simulink model "IMFaults"  (R2025b)
settings: Solver=ode23t  StartTime=0.0  StopTime=20  MaxStep=1e-4  RelTol=1e-3  EnableMultiTasking=on
undefined symbols (not defined in the file or in its folder): DELTA_A, DELTA_B, DELTA_C, V_phase
libraries: ee_lib x13, nesl_utility x10, fl_lib x9
CloseFcn:
  | clear simlog_IMStarting
  | clear logsout_IMStarting
Description:
  | Three-Phase Asynchronous Machine Starting
settings Model: Creator=The MathWorks, Inc.  LastModifiedBy=Hp Probook
settings SolverCC: AlgebraicLoopSolver=TrustRegion  MaxZcPerStep=1.0
settings DataIOCC: LimitDataPoints=on  MaxDataPoints=90000  SaveFormat=Array  ReturnWorkspaceOutputs=off
settings OptimizationCC: ReuseModelBlockBuffer=off  LifeSpan=inf
settings DebuggingCC: UnconnectedInputMsg=warning  UnconnectedOutputMsg=warning  UnconnectedLineMsg=warning  SFUnexpectedBacktrackingDiag=warning  SFNoUnconditionalDefaultTransitionDiag=warning  SFExecutionAtInitializationDiag=none  ArithmeticOperatorsInVariantConditions=warning
settings HardwareCC: ProdBitPerPointer=32.0  ProdBitPerSizeT=32.0  ProdBitPerPtrDiffT=32.0  ProdLargestAtomicFloat=None  ProdIntDivRoundTo=Undefined  ProdEndianess=Unspecified  ProdWordSize=32.0  ProdHWDeviceType=32-bit Generic
settings ModelReferenceCC: EnableRefExpFcnMdlSchedulingChecks=on  PropagateSignalLabelsOutOfModel=off
settings SFSimCC: SimUseLocalCustomCode=off  CustomCodeUndefinedFunction=UseInterfaceOnly
settings RTWCC: RTWUseLocalCustomCode=off  GPUComputeCapability=3.5  DLArmComputeVersion=19.05
settings CodeAppCC: StateflowObjectComments=on
settings GRTTargetCC: TargetLangStandard=C89/C90 (ANSI)
settings ConfigComp: CovMetricSettings=dw  CovSaveCumulativeToWorkspaceVar=on  CovSaveSingleToWorkspaceVar=on  CovExternalEMLEnable=off  CovSFcnEnable=off
settings SimscapeCC: SimscapeLogType=all  SimscapeLogSimulationStatistics=on  SimscapeLogName=simlog_IMStarting  SimscapeLogDataHistory=90000.0

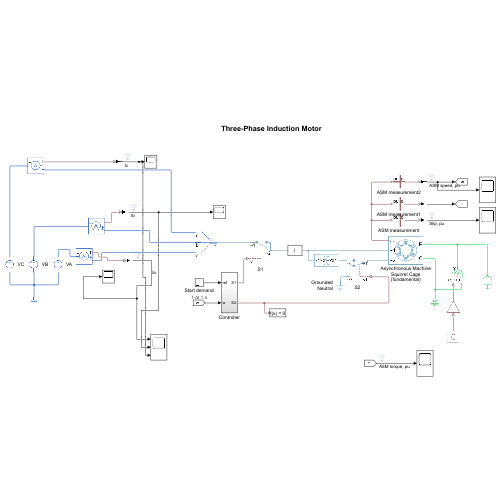
[thumbnail: Simulink's stored preview of the top-level diagram]
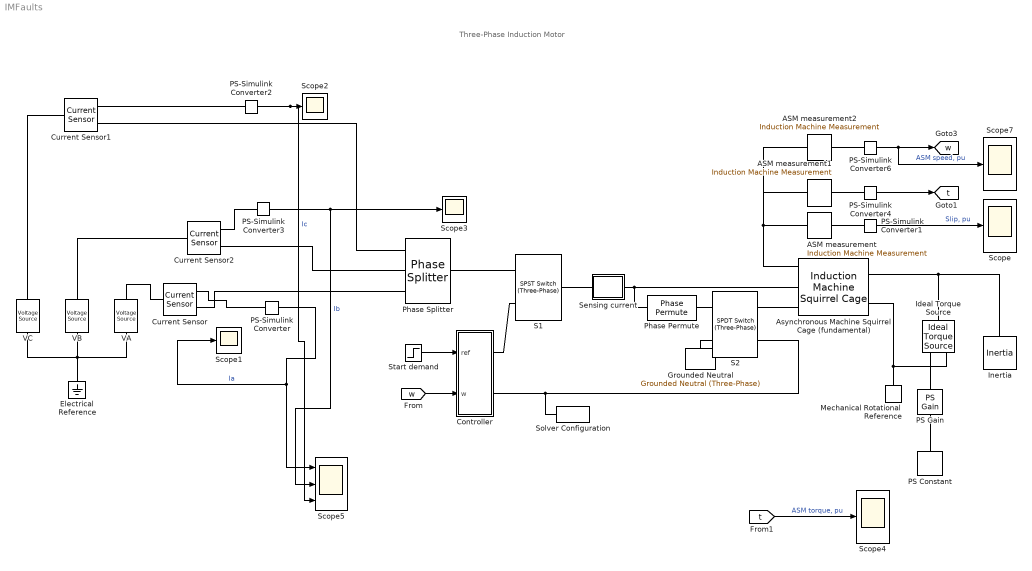
== system IMFaults ==
  note: Three-Phase Induction Motor
  ASM measurement : ee_lib/Electromechanical/Asynchronous/Induction Machine Measurement  output_idx=9
      settings: InternalSimscapePortConfiguration="{\"Bottom\":[],\"Left\":[{\"id\":\"pu_input\",\"label\":\"pu\",\"type\":\"input\"}],\"Right\":[{\"id\":\"pu_output\",\"label\":\"o\",\"type\":\"output\"}],\"Top\":[]}"
  ASM measurement1 : ee_lib/Electromechanical/Asynchronous/Induction Machine Measurement  output_idx=1
      settings: InternalSimscapePortConfiguration="{\"Bottom\":[],\"Left\":[{\"id\":\"pu_input\",\"label\":\"pu\",\"type\":\"input\"}],\"Right\":[{\"id\":\"pu_output\",\"label\":\"o\",\"type\":\"output\"}],\"Top\":[]}"
  ASM measurement2 : ee_lib/Electromechanical/Asynchronous/Induction Machine Measurement  output_idx=2
      settings: InternalSimscapePortConfiguration="{\"Bottom\":[],\"Left\":[{\"id\":\"pu_input\",\"label\":\"pu\",\"type\":\"input\"}],\"Right\":[{\"id\":\"pu_output\",\"label\":\"o\",\"type\":\"output\"}],\"Top\":[]}"
  Asynchronous Machine Squirrel Cage (fundamental) : ee_lib/Electromechanical/Asynchronous/Induction Machine Squirrel Cage  port_option=ee.enum.threePhasePort.composite  SRated=15e3 V*A  VRated=220 V  FRated=60 Hz  nPolePairs=1  param_unit=ee.enum.unit.pu  squirrel_cage=ee.enum.squirrelcage.Single  zero_sequence=ee.enum.park.zerosequence.include  initialization_option=ee.enum.asm.initialization.fluxvariables  Rs=0.25 Ohm  Xls=0.4 Ohm  pu_Rs=0.0258  pu_Lls=0.0413  Rrd=0.14 Ohm  Xlrd=0.41 Ohm  pu_Rrd=0.0145  pu_Llrd=0.0424  Rrd1=0.28 Ohm  Xlrd1=0.82 Ohm  Rrd2=0.28 Ohm  Xlrd2=0.82 Ohm  pu_Rrd1=0.0290  pu_Llrd1=0.0848  pu_Rrd2=0.0290  pu_Llrd2=0.0848  Xm=17 Ohm  pu_Lm=1.7562  X0=0.4 Ohm  pu_L0=0.0413  saturation_option=ee.enum.saturation.include  saturation_i=[0, 4, 9, 18, 25, 34, 50, 68, 95, 120] A  saturation_v=[0, 88, 154, 198, 220, 242, 264, 286, 308, 327] V  pu_saturation_i=[0, .176, .396, .792, 1.1, 1.496, 2.2, 2.992, 4.18, 5.28]  pu_saturation_v=[0, .4, .7, .9, 1, 1.1, 1.2, 1.3, 1.4, 1.4864]  connection_option=ee.enum.Connection.delta1  angular_position_specify=off  angular_position_priority=None  angular_position=0 deg  angular_position_nominal_specify=off  angular_position_nominal_value=1  angular_position_nominal_unit=deg  pu_psids_specify=off  pu_psids_priority=None  pu_psids=0  pu_psids_nominal_specify=off  pu_psids_nominal_value=1  pu_psids_nominal_unit=1  pu_psiqs_specify=off  pu_psiqs_priority=None  pu_psiqs=0  pu_psiqs_nominal_specify=off  pu_psiqs_nominal_value=1  pu_psiqs_nominal_unit=1  pu_psi0s_specify=off  pu_psi0s_priority=None  pu_psi0s=0  pu_psi0s_nominal_specify=off  pu_psi0s_nominal_value=1  pu_psi0s_nominal_unit=1  pu_psidr_specify=off  pu_psidr_priority=None  pu_psidr=0  pu_psidr_nominal_specify=off  pu_psidr_nominal_value=1  pu_psidr_nominal_unit=1  pu_psiqr_specify=off  pu_psiqr_priority=None  pu_psiqr=0  pu_psiqr_nominal_specify=off  pu_psiqr_nominal_value=1  pu_psiqr_nominal_unit=1  pu_psidr1_specify=off  pu_psidr1_priority=None  pu_psidr1=0  pu_psidr1_nominal_specify=off  pu_psidr1_nominal_value=1  pu_psidr1_nominal_unit=1  pu_psiqr1_specify=off  pu_psiqr1_priority=None  pu_psiqr1=0  pu_psiqr1_nominal_specify=off  pu_psiqr1_nominal_value=1  pu_psiqr1_nominal_unit=1  pu_psidr2_specify=off  pu_psidr2_priority=None  pu_psidr2=0  pu_psidr2_nominal_specify=off  pu_psidr2_nominal_value=1  pu_psidr2_nominal_unit=1  pu_psiqr2_specify=off  pu_psiqr2_priority=None  pu_psiqr2=0  pu_psiqr2_nominal_specify=off  pu_psiqr2_nominal_value=1  pu_psiqr2_nominal_unit=1  psids_specify=off  psids_priority=None  psids=0 Wb  psids_nominal_specify=off  psids_nominal_value=1  psids_nominal_unit=Wb  psiqs_specify=off  psiqs_priority=None  psiqs=0 Wb  psiqs_nominal_specify=off  psiqs_nominal_value=1  psiqs_nominal_unit=Wb  psi0s_specify=off  psi0s_priority=None  psi0s=0 Wb  psi0s_nominal_specify=off  psi0s_nominal_value=1  psi0s_nominal_unit=Wb  psidr_specify=off  psidr_priority=None  psidr=0 Wb  psidr_nominal_specify=off  psidr_nominal_value=1  psidr_nominal_unit=Wb  psiqr_specify=off  psiqr_priority=None  psiqr=0 Wb  psiqr_nominal_specify=off  psiqr_nominal_value=1  psiqr_nominal_unit=Wb  psidr1_specify=off  psidr1_priority=None  psidr1=0 Wb  psidr1_nominal_specify=off  psidr1_nominal_value=1  psidr1_nominal_unit=Wb  psiqr1_specify=off  psiqr1_priority=None  psiqr1=0 Wb  psiqr1_nominal_specify=off  psiqr1_nominal_value=1  psiqr1_nominal_unit=Wb  psidr2_specify=off  psidr2_priority=None  psidr2=0 Wb  psidr2_nominal_specify=off  psidr2_nominal_value=1  psidr2_nominal_unit=Wb  psiqr2_specify=off  psiqr2_priority=None  psiqr2=0 Wb  psiqr2_nominal_specify=off  psiqr2_nominal_value=1  psiqr2_nominal_unit=Wb  slip_specify=off  slip_priority=None  slip=0  slip_nominal_specify=off  slip_nominal_value=1  slip_nominal_unit=1  real_power_generated_specify=off  real_power_generated_priority=None  real_power_generated=0 W  real_power_generated_nominal_specify=off  real_power_generated_nominal_value=1  real_power_generated_nominal_unit=W  mechanical_power_consumed_specify=off  mechanical_power_consumed_priority=None  mechanical_power_consumed=0 W  mechanical_power_consumed_nominal_specify=off  mechanical_power_consumed_nominal_value=1  mechanical_power_consumed_nominal_unit=W  Tmeas=298.15 K  alpha=3.93e-3 1/K  alpha_cage=4.4e-3 1/K  stator_thermal_mass=100 J/K  rotor_thermal_mass=200 J/K  temperatureA_specify=off  temperatureA_priority=High  temperatureA=25 degC  temperatureA_nominal_specify=off  temperatureA_nominal_value=1  temperatureA_nominal_unit=degC  temperatureB_specify=off  temperatureB_priority=High  temperatureB=25 degC  temperatureB_nominal_specify=off  temperatureB_nominal_value=1  temperatureB_nominal_unit=degC  temperatureC_specify=off  temperatureC_priority=High  temperatureC=25 degC  temperatureC_nominal_specify=off  temperatureC_nominal_value=1  temperatureC_nominal_unit=degC  temperatureR_specify=off  temperatureR_priority=High  temperatureR=25 degC  temperatureR_nominal_specify=off  temperatureR_nominal_value=1  temperatureR_nominal_unit=degC
      settings: InternalSimscapePortConfiguration="{\"Bottom\":[],\"Left\":[{\"id\":\"R\",\"label\":\"R\",\"type\":\"foundation.mechanical.rotational.rotational\"},{\"id\":\"C\",\"label\":\"C\",\"type\":\"foundation.mechanical.rotational.rotational\"}],\"Right\":[{\"id\":\"pu_output\",\"label\":\"pu\",\"type\":\"output\"},{\"id\":\"N1\",\"label\":\"~1\",\"type\":\"foundation.electrical.three_phase\"},{\"id\":\"N2\",\"label\":\"~2\",\"type\":\"foundation.electrical.three_phase\"}],\"Top\":[]}"
  Controller : Subsystem
  Current Sensor : fl_lib/Electrical/Electrical Sensors/Current Sensor
  Current Sensor1 : fl_lib/Electrical/Electrical Sensors/Current Sensor
  Current Sensor2 : fl_lib/Electrical/Electrical Sensors/Current Sensor
  Electrical Reference : fl_lib/Electrical/Electrical Elements/Electrical Reference
  Grounded Neutral : ee_lib/Connectors & References/Grounded Neutral (Three-Phase)
  Ideal Torque Source : fl_lib/Mechanical/Mechanical Sources/Ideal Torque Source
  Inertia : fl_lib/Mechanical/Rotational Elements/Inertia  inertia=0.001 kg*m^2  num_ports=foundation.enum.numPorts2.one  w_specify=off  w_priority=High  w=0 rad/s  w_nominal_specify=off  w_nominal_value=1  w_nominal_unit=rad/s  t_specify=off  t_priority=None  t=0 N*m  t_nominal_specify=off  t_nominal_value=1  t_nominal_unit=N*m
  Mechanical Rotational Reference : fl_lib/Mechanical/Rotational Elements/Mechanical Rotational Reference
  PS Constant : fl_lib/Physical Signals/Sources/PS Constant  constant=10 N*m
  PS Gain : fl_lib/Physical Signals/Functions/PS Gain  gain=-2
  PS-Simulink Converter : nesl_utility/PS-Simulink Converter  PhysicalDomain=network_engine_domain  SubClassName=ps_output  LeftPortType=input  RightPortType=output  PseudoPeriodic=off  Frequencies=[]  VectorFormat=inherit  Unit=inherit  AffineConversion=off
  PS-Simulink Converter1 : nesl_utility/PS-Simulink Converter  PhysicalDomain=network_engine_domain  SubClassName=ps_output  LeftPortType=input  RightPortType=output  PseudoPeriodic=off  Frequencies=[]  VectorFormat=1-D array  Unit=1  AffineConversion=off
  PS-Simulink Converter2 : nesl_utility/PS-Simulink Converter  PhysicalDomain=network_engine_domain  SubClassName=ps_output  LeftPortType=input  RightPortType=output  PseudoPeriodic=off  Frequencies=[]  VectorFormat=inherit  Unit=inherit  AffineConversion=off
  PS-Simulink Converter3 : nesl_utility/PS-Simulink Converter  PhysicalDomain=network_engine_domain  SubClassName=ps_output  LeftPortType=input  RightPortType=output  PseudoPeriodic=off  Frequencies=[]  VectorFormat=inherit  Unit=inherit  AffineConversion=off
  PS-Simulink Converter4 : nesl_utility/PS-Simulink Converter  PhysicalDomain=network_engine_domain  SubClassName=ps_output  LeftPortType=input  RightPortType=output  PseudoPeriodic=off  Frequencies=[]  VectorFormat=1-D array  Unit=1  AffineConversion=off
  PS-Simulink Converter6 : nesl_utility/PS-Simulink Converter  PhysicalDomain=network_engine_domain  SubClassName=ps_output  LeftPortType=input  RightPortType=output  PseudoPeriodic=off  Frequencies=[]  VectorFormat=1-D array  Unit=1  AffineConversion=off
  Phase Permute : ee_lib/Connectors & References/Phase Permute
      settings: InternalSimscapePortConfiguration="{\"Bottom\":[],\"Left\":[{\"id\":\"N123\",\"label\":\"~123\",\"type\":\"foundation.electrical.three_phase\"}],\"Right\":[{\"id\":\"N231\",\"label\":\"~231\",\"type\":\"foundation.electrical.three_phase\"}],\"Top\":[]}"
  Phase Splitter : ee_lib/Connectors & References/Phase Splitter
  S1 : ee_lib/Switches & Breakers/SPST Switch (Three-Phase)  R_closed=0.001 Ohm  G_open=1e-6 1/Ohm  threshold=0.5 V  i_vT_specify=off  i_vT_priority=None  i_vT=0 A  i_vT_nominal_specify=off  i_vT_nominal_value=1  i_vT_nominal_unit=A  I_specify=off  I_priority=None  I=[ 0 0 0 ] A  I_nominal_specify=off  I_nominal_value=1  I_nominal_unit=A  V_specify=off  V_priority=None  V=[ 0 0 0 ] V  V_nominal_specify=off  V_nominal_value=1  V_nominal_unit=V  i_a_specify=off  i_a_priority=None  i_a=0 A  i_a_nominal_specify=off  i_a_nominal_value=1  i_a_nominal_unit=A  v_a_specify=off  v_a_priority=None  v_a=0 V  v_a_nominal_specify=off  v_a_nominal_value=1  v_a_nominal_unit=V  i_b_specify=off  i_b_priority=None  i_b=0 A  i_b_nominal_specify=off  i_b_nominal_value=1  i_b_nominal_unit=A  v_b_specify=off  v_b_priority=None  v_b=0 V  v_b_nominal_specify=off  v_b_nominal_value=1  v_b_nominal_unit=V  i_c_specify=off  i_c_priority=None  i_c=0 A  i_c_nominal_specify=off  i_c_nominal_value=1  i_c_nominal_unit=A  v_c_specify=off  v_c_priority=None  v_c=0 V  v_c_nominal_specify=off  v_c_nominal_value=1  v_c_nominal_unit=V
      settings: InternalSimscapePortConfiguration="{\"Bottom\":[],\"Left\":[{\"id\":\"vT\",\"label\":\"vT\",\"type\":\"input\"},{\"id\":\"N1\",\"label\":\"~1\",\"type\":\"foundation.electrical.three_phase\"}],\"Right\":[{\"id\":\"N2\",\"label\":\"~2\",\"type\":\"foundation.electrical.three_phase\"}],\"Top\":[]}"
  S2 : ee_lib/Switches & Breakers/SPDT Switch (Three-Phase)  R_closed=0.001 Ohm  G_open=1e-6 1/Ohm  threshold=0.5 V  i_vT_specify=off  i_vT_priority=None  i_vT=0 A  i_vT_nominal_specify=off  i_vT_nominal_value=1  i_vT_nominal_unit=A  I12_specify=off  I12_priority=None  I12=[ 0 0 0 ] A  I12_nominal_specify=off  I12_nominal_value=1  I12_nominal_unit=A  V12_specify=off  V12_priority=None  V12=[ 0 0 0 ] V  V12_nominal_specify=off  V12_nominal_value=1  V12_nominal_unit=V  I13_specify=off  I13_priority=None  I13=[ 0 0 0 ] A  I13_nominal_specify=off  I13_nominal_value=1  I13_nominal_unit=A  V13_specify=off  V13_priority=None  V13=[ 0 0 0 ] V  V13_nominal_specify=off  V13_nominal_value=1  V13_nominal_unit=V  i_a_12_specify=off  i_a_12_priority=None  i_a_12=0 A  i_a_12_nominal_specify=off  i_a_12_nominal_value=1  i_a_12_nominal_unit=A  v_a_12_specify=off  v_a_12_priority=None  v_a_12=0 V  v_a_12_nominal_specify=off  v_a_12_nominal_value=1  v_a_12_nominal_unit=V  i_a_13_specify=off  i_a_13_priority=None  i_a_13=0 A  i_a_13_nominal_specify=off  i_a_13_nominal_value=1  i_a_13_nominal_unit=A  v_a_13_specify=off  v_a_13_priority=None  v_a_13=0 V  v_a_13_nominal_specify=off  v_a_13_nominal_value=1  v_a_13_nominal_unit=V  i_b_12_specify=off  i_b_12_priority=None  i_b_12=0 A  i_b_12_nominal_specify=off  i_b_12_nominal_value=1  i_b_12_nominal_unit=A  v_b_12_specify=off  v_b_12_priority=None  v_b_12=0 V  v_b_12_nominal_specify=off  v_b_12_nominal_value=1  v_b_12_nominal_unit=V  i_b_13_specify=off  i_b_13_priority=None  i_b_13=0 A  i_b_13_nominal_specify=off  i_b_13_nominal_value=1  i_b_13_nominal_unit=A  v_b_13_specify=off  v_b_13_priority=None  v_b_13=0 V  v_b_13_nominal_specify=off  v_b_13_nominal_value=1  v_b_13_nominal_unit=V  i_c_12_specify=off  i_c_12_priority=None  i_c_12=0 A  i_c_12_nominal_specify=off  i_c_12_nominal_value=1  i_c_12_nominal_unit=A  v_c_12_specify=off  v_c_12_priority=None  v_c_12=0 V  v_c_12_nominal_specify=off  v_c_12_nominal_value=1  v_c_12_nominal_unit=V  i_c_13_specify=off  i_c_13_priority=None  i_c_13=0 A  i_c_13_nominal_specify=off  i_c_13_nominal_value=1  i_c_13_nominal_unit=A  v_c_13_specify=off  v_c_13_priority=None  v_c_13=0 V  v_c_13_nominal_specify=off  v_c_13_nominal_value=1  v_c_13_nominal_unit=V
      settings: InternalSimscapePortConfiguration="{\"Bottom\":[],\"Left\":[{\"id\":\"vT\",\"label\":\"vT\",\"type\":\"input\"},{\"id\":\"N1\",\"label\":\"~1\",\"type\":\"foundation.electrical.three_phase\"}],\"Right\":[{\"id\":\"N2\",\"label\":\"~2\",\"type\":\"foundation.electrical.three_phase\"},{\"id\":\"N3\",\"label\":\"~3\",\"type\":\"foundation.electrical.three_phase\"}],\"Top\":[]}"
  Scope{,1..4,7} (6 alike) : Scope
      Scope settings: ActiveDisplayYMinimum=-64.774660970557036  ActiveDisplayYMaximum=592.97194873501348  DataLoggingVariableName=log_slip
      Scope1 settings: TimeSpan=1.5  ActiveDisplayYMinimum=-580.942172059893  ActiveDisplayYMaximum=426.13053331341985
      Scope2 settings: TimeSpan=0.7  ActiveDisplayYMinimum=-299.05789642595164  ActiveDisplayYMaximum=375.59644921938911  DataLoggingVariableName=ScopeData2
      Scope3 settings: TimeSpan=2  ActiveDisplayYMinimum=-316.27067649423543  ActiveDisplayYMaximum=308.17944764779912  DataLoggingVariableName=ScopeData3
      Scope4 settings: ActiveDisplayYMinimum=-1245.0608675400504  ActiveDisplayYMaximum=1413.8796251256649  DataLoggingVariableName=log_electrical_torque
      Scope7 settings: ActiveDisplayYMinimum=-3976.0404220166  ActiveDisplayYMaximum=3972.2451291285806  DataLoggingVariableName=log_speed
  Scope5 : Scope  NumInputPorts=3
      settings: ActiveDisplayYMinimum=-358.01728461363564  ActiveDisplayYMaximum=364.75896133338756  DataLoggingVariableName=log_currents
  Sensing current : Subsystem
      mask Display: disp('i')
  Solver Configuration : nesl_utility/Solver Configuration  PhysicalDomain=network_engine_domain  SubClassName=solver  LeftPortType=input  RightPortType=generic  Tones=[]  Harmonics=[]  SimulateNoise=off  Profile=off  UseLocalSampling=off  EnableSwitchedLinearOptims=on  FrequencyDomain=off  UseCCode=off  RelTol=0.001  AbsTol=1e-06  MinStep=1e-09  ToWorkspace=off  RevertToSquareIcSolve=off  NumHomotopyIterations=100  PhasorMode=off  PhasorModeNumHarmonics=1  ConsistencySolver=NEWTON_FTOL  IndexReductionMethod=DerivativeReplacement  DoDC=off  ResidualTolerance=1e-9  ConsistencyTolSource=GLOBAL  ConsistencyAbsTol=0.001  ConsistencyRelTol=0.001  ConsistencyTolFactor=0.001  UseLocalSolver=off  LocalSolverChoice=NE_BACKWARD_EULER_ADVANCER  ResolveIndetEquations=on  FunctionEvalNumThread=1  LocalSolverSampleTime=1e-4  DoFixedCost=off  MaxNonlinIter=3  MaxModeIter=2  ComputeImpulses=off  ImpulseIterations=2  LinearAlgebra=auto  LinearAlgebraNumThread=0  EquationFormulation=NE_TIME_EF  DelaysMemoryBudget=1024  AutomaticFiltering=on  FilteringTimeConstant=0.001  PartitionStorageMethod=AS_NEEDED  PartitionMemoryBudget=1024  PartitionMethod=FAST  MultibodyUseLocalSolver=off  MultibodyLocalSolverChoice=ODE1  MultibodyLocalSolverSampleTime=0.001
  Start demand : Step  SampleTime=0
      settings: AttributesFormatString=%<After> at %<Time> s
  VA : ee_lib/Sources/Voltage Source  dc_voltage=0 V  ac_voltage=|  ac_shift=0 rad  ac_frequency=60 Hz  noise_mode=ee.enum.sources.noise.Disabled  PSD=0 V^2/Hz  sample_time=1e-3 s  repeatability=ee.enum.sources.repeatability.NotRepeatable  user_seed=0  auto_seed=3499211588  i_specify=off  i_priority=None  i=0 A  i_nominal_specify=off  i_nominal_value=1  i_nominal_unit=A  v_specify=off  v_priority=None  v=0 V  v_nominal_specify=off  v_nominal_value=1  v_nominal_unit=V
      | V_phase * (1 + DELTA_A)
      |  V
  VB : ee_lib/Sources/Voltage Source  dc_voltage=0 V  ac_voltage=|  ac_shift=-120 deg  ac_frequency=60 Hz  noise_mode=ee.enum.sources.noise.Disabled  PSD=0 V^2/Hz  sample_time=1e-3 s  repeatability=ee.enum.sources.repeatability.NotRepeatable  user_seed=0  auto_seed=3890346746  i_specify=off  i_priority=None  i=0 A  i_nominal_specify=off  i_nominal_value=1  i_nominal_unit=A  v_specify=off  v_priority=None  v=0 V  v_nominal_specify=off  v_nominal_value=1  v_nominal_unit=V
      | V_phase * (1 + DELTA_B)
      |  V
  VC : ee_lib/Sources/Voltage Source  dc_voltage=0 V  ac_voltage=|  ac_shift=120 deg  ac_frequency=60 Hz  noise_mode=ee.enum.sources.noise.Disabled  PSD=0 V^2/Hz  sample_time=1e-3 s  repeatability=ee.enum.sources.repeatability.NotRepeatable  user_seed=0  auto_seed=545404223  i_specify=off  i_priority=None  i=0 A  i_nominal_specify=off  i_nominal_value=1  i_nominal_unit=A  v_specify=off  v_priority=None  v=0 V  v_nominal_specify=off  v_nominal_value=1  v_nominal_unit=V
      | V_phase * (1 + DELTA_C)
      |  V
  tag scope: t=global, w=global
  wires:
  Start demand/1 -> Controller/1(ref)
  PS-Simulink Converter1/1 -> Scope/1  "Slip, pu"
  PS-Simulink Converter/1 -> Scope5/1, Scope1/1  "Ia"
  PS-Simulink Converter2/1 -> Scope5/3, Scope2/1  "Ic"
  PS-Simulink Converter3/1 -> Scope5/2, Scope3/1  "Ib"
  [t] -> Scope4/1  "ASM torque, pu"
  PS-Simulink Converter4/1 -> [t]
  PS-Simulink Converter6/1 -> Scope7/1, [w]  "ASM speed, pu"
  [w] -> Controller/2(w)
  connections:
  Sensing current/RConn1 -- Asynchronous Machine Squirrel Cage (fundamental)/RConn2 -- Phase Permute/LConn1
  S2/LConn2 -- Asynchronous Machine Squirrel Cage (fundamental)/RConn3
  S2/RConn1 -- Grounded Neutral/LConn1
  Controller/RConn1 -- S1/LConn1
  Controller/RConn2 -- S2/LConn1 -- Solver Configuration/RConn1
  Asynchronous Machine Squirrel Cage (fundamental)/RConn1 -- ASM measurement2/LConn1 -- ASM measurement1/LConn1 -- ASM measurement/LConn1
  ASM measurement/RConn1 -- PS-Simulink Converter1/LConn1
  Phase Permute/RConn1 -- S2/RConn2
  S1/RConn1 -- Sensing current/LConn1
  Phase Splitter/LConn1 -- S1/LConn2
  VA/RConn1 -- VC/RConn1 -- Electrical Reference/LConn1 -- VB/RConn1
  VA/LConn1 -- Current Sensor/LConn1
  Phase Splitter/RConn1 -- Current Sensor/RConn2
  Current Sensor/RConn1 -- PS-Simulink Converter/LConn1
  VC/LConn1 -- Current Sensor1/LConn1
  VB/LConn1 -- Current Sensor2/LConn1
  PS-Simulink Converter3/LConn1 -- Current Sensor2/RConn1
  Phase Splitter/RConn2 -- Current Sensor2/RConn2
  Current Sensor1/RConn2 -- Phase Splitter/RConn3
  Current Sensor1/RConn1 -- PS-Simulink Converter2/LConn1
  Inertia/LConn1 -- Asynchronous Machine Squirrel Cage (fundamental)/LConn1 -- Ideal Torque Source/LConn1
  Asynchronous Machine Squirrel Cage (fundamental)/LConn2 -- Ideal Torque Source/RConn2 -- Mechanical Rotational Reference/LConn1
  ASM measurement1/RConn1 -- PS-Simulink Converter4/LConn1
  ASM measurement2/RConn1 -- PS-Simulink Converter6/LConn1
  PS Gain/RConn1 -- Ideal Torque Source/RConn1
  PS Gain/LConn1 -- PS Constant/RConn1

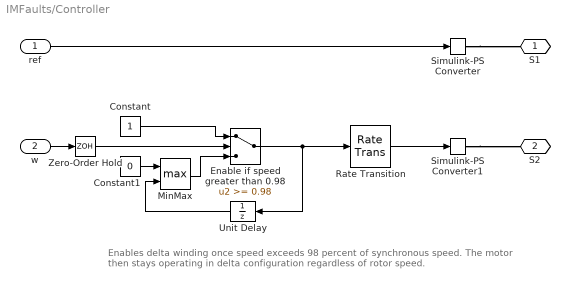
== system IMFaults/Controller ==
  note: Enables delta winding once speed exceeds 98 percent of synchronous
      | speed. The motor then stays operating in delta configuration regardless
      | of rotor speed.
  ref : Inport
  w : Inport  Port=2
  Constant : Constant
  Constant1 : Constant  Value=0
  Enable if speed greater than 0.98 : Switch  Threshold=0.98  SaturateOnIntegerOverflow=off  InputSameDT=off
  MinMax : MinMax  Function=max  Inputs=2
  Rate Transition : RateTransition
  Simulink-PS Converter : nesl_utility/Simulink-PS Converter  PhysicalDomain=network_engine_domain  SubClassName=ps_input  LeftPortType=input  RightPortType=output  PseudoPeriodic=off  Frequencies=[]  NoiseDistribution=none  NoiseParameters=[]  Unit=1  AffineConversion=off  FilteringAndDerivatives=zero  SimscapeFilterOrder=1  InputFilterTimeConstant=0.001  UdotUserProvided=1
  Simulink-PS Converter1 : nesl_utility/Simulink-PS Converter  PhysicalDomain=network_engine_domain  SubClassName=ps_input  LeftPortType=input  RightPortType=output  PseudoPeriodic=off  Frequencies=[]  NoiseDistribution=none  NoiseParameters=[]  Unit=1  AffineConversion=off  FilteringAndDerivatives=zero  SimscapeFilterOrder=1  InputFilterTimeConstant=0.001  UdotUserProvided=1
  Unit Delay : UnitDelay  SampleTime=0.1  HasFrameUpgradeWarning=on
  Zero-Order Hold : ZeroOrderHold  SampleTime=0.1
  S1 : PMIOPort  Side=Right
  S2 : PMIOPort  Port=2  Side=Right
  wires:
  ref/1 -> Simulink-PS Converter/1
  Enable if speed greater than 0.98/1 -> Unit Delay/1, Rate Transition/1
  Constant/1 -> Enable if speed greater than 0.98/1
  w/1 -> Zero-Order Hold/1
  Zero-Order Hold/1 -> Enable if speed greater than 0.98/2
  Rate Transition/1 -> Simulink-PS Converter1/1
  MinMax/1 -> Enable if speed greater than 0.98/3
  Constant1/1 -> MinMax/1
  Unit Delay/1 -> MinMax/2
  connections:
  Simulink-PS Converter/RConn1 -- S1/RConn1
  Simulink-PS Converter1/RConn1 -- S2/RConn1

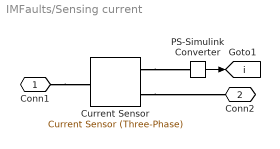
== system IMFaults/Sensing current ==
  Current Sensor : ee_lib/Sensors & Transducers/Current Sensor (Three-Phase)
  PS-Simulink Converter : nesl_utility/PS-Simulink Converter  PhysicalDomain=network_engine_domain  SubClassName=ps_output  LeftPortType=input  RightPortType=output  PseudoPeriodic=off  Frequencies=[]  VectorFormat=1-D array  Unit=1  AffineConversion=off
  Conn1 : PMIOPort  Side=Left
  Conn2 : PMIOPort  Port=2  Side=Right
  tag scope: i=global
  wires:
  PS-Simulink Converter/1 -> [i]
  connections:
  Current Sensor/RConn1 -- PS-Simulink Converter/LConn1
  Conn1/RConn1 -- Current Sensor/LConn1
  Current Sensor/RConn2 -- Conn2/RConn1
